simulink model "gen"  (Simulink 7.5)
settings: Solver=ode45  StartTime=0.0  StopTime=10.0  RelTol=1e-3
settings Model: Creator=sisa  LastModifiedBy=SISA

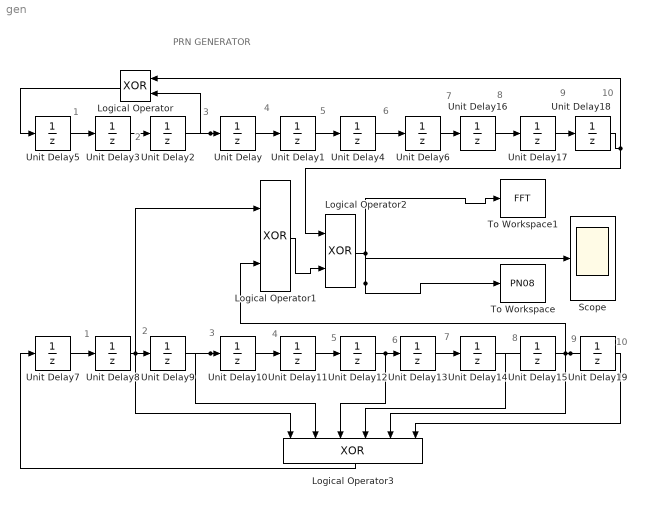
== system gen ==
  note: 1
  note: 2
  note: 3
  note: 4
  note: 5
  note: 6
  note: 7
  note: 8
  note: 9
  note: 10
  note: PRN GENERATOR
  note: 1
  note: 2
  note: 3
  note: 4
  note: 5
  note: 6
  note: 7
  note: 8
  note: 9
  note: 10
  Logical Operator : Logic  Operator=XOR  AllPortsSameDT=off  OutDataTypeMode=boolean  LogicDataType=fixdt(0, 8)  OutDataTypeStr=boolean
  Logical Operator1 : Logic  Operator=XOR  AllPortsSameDT=off  OutDataTypeMode=boolean  LogicDataType=fixdt(0, 8)  OutDataTypeStr=boolean
  Logical Operator2 : Logic  Operator=XOR  AllPortsSameDT=off  OutDataTypeMode=boolean  LogicDataType=fixdt(0, 8)  OutDataTypeStr=boolean
  Logical Operator3 : Logic  Operator=XOR  Inputs=6  AllPortsSameDT=off  OutDataTypeMode=boolean  LogicDataType=fixdt(0, 8)  OutDataTypeStr=boolean
  Scope : Scope
      settings: TimeRange=10  SampleInput=on
  To Workspace : ToWorkspace  VariableName=PN08  SampleTime=-1  SaveFormat=Array
      settings: MaxDataPoints=1023000
  To Workspace1 : ToWorkspace  VariableName=FFT  SampleTime=-1  SaveFormat=Array
      settings: MaxDataPoints=1023000
  Unit Delay{,1..19} (20 alike) : UnitDelay  X0=1  SampleTime=-1
  wires:
  Unit Delay3/1 -> Unit Delay2/1
  Unit Delay2/1 -> Unit Delay/1, Logical Operator/2
  Unit Delay/1 -> Unit Delay1/1
  Unit Delay1/1 -> Unit Delay4/1
  Unit Delay5/1 -> Unit Delay3/1
  Unit Delay4/1 -> Unit Delay6/1
  Unit Delay6/1 -> Unit Delay16/1
  Unit Delay16/1 -> Unit Delay17/1
  Unit Delay17/1 -> Unit Delay18/1
  Unit Delay7/1 -> Unit Delay8/1
  Unit Delay9/1 -> Logical Operator3/2, Unit Delay10/1
  Unit Delay10/1 -> Unit Delay11/1
  Unit Delay11/1 -> Unit Delay12/1
  Unit Delay12/1 -> Logical Operator3/3, Unit Delay13/1
  Unit Delay13/1 -> Unit Delay14/1
  Unit Delay14/1 -> Logical Operator3/4, Unit Delay15/1
  Unit Delay15/1 -> Unit Delay19/1, Logical Operator3/5, Logical Operator1/2
  Logical Operator/1 -> Unit Delay5/1
  Logical Operator2/1 -> Scope/1, To Workspace/1, To Workspace1/1
  Unit Delay18/1 -> Logical Operator2/1, Logical Operator/1
  Logical Operator1/1 -> Logical Operator2/2
  Logical Operator3/1 -> Unit Delay7/1
  Unit Delay19/1 -> Logical Operator3/6
  Unit Delay8/1 -> Logical Operator3/1, Unit Delay9/1, Logical Operator1/1
